simulink model "otonom_sim"  (R2021b)
settings: Solver=VariableStepAuto  StartTime=0.0  StopTime=50  RelTol=1e-3
libraries: sim3dautolib x2, slpidlib x1, robotmobilelib x1, simulink x1, sim3dlib x1
settings Model: Creator=Asus  LastModifiedBy=cx

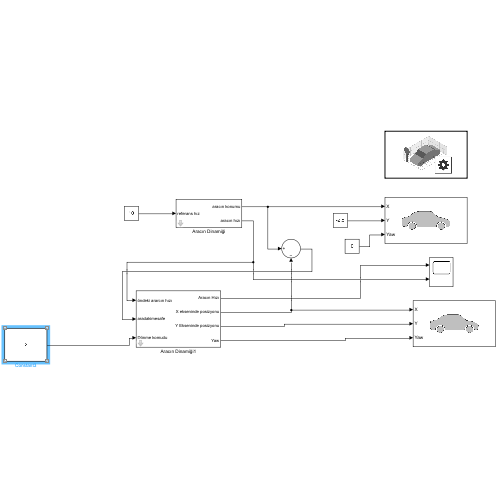
[thumbnail: Simulink's stored preview of the top-level diagram]
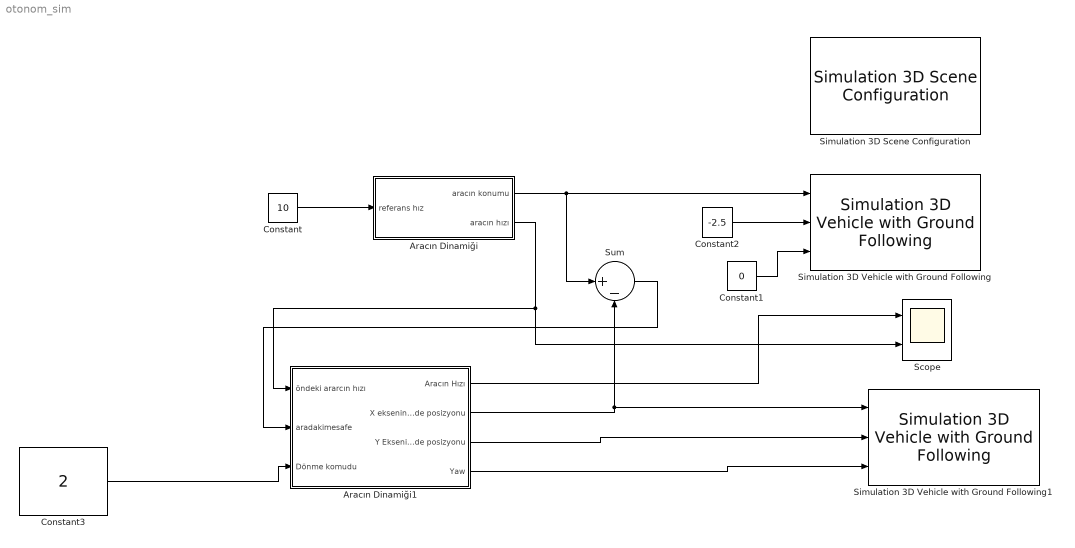
== system otonom_sim ==
  Aracın Dinamiği : Subsystem  mask{Konum=40, Hiz=20}
      mask prompts: Konum "Başlangıç Konumu"; Hiz "Başlangıç Hızı"
      mask TypeOptions Konum: başlangıç konumu/Value
      mask TypeOptions Hiz: başlangıç hızı/Value
  Aracın Dinamiği1 : Subsystem  mask{Konum=20, Hiz=40}
      mask prompts: Konum "Başlangıç Konumu"; Hiz "Başlangıç Hızı"
      mask TypeOptions Konum: başlangıç konumu/Value
      mask TypeOptions Hiz: başlangıç hızı/Value
  Constant : Constant  Value=10
  Constant1 : Constant  Value=0
  Constant2 : Constant  Value=-2.5
  Constant3 : Constant  Value=2
  Scope : Scope  NumInputPorts=2
  Simulation 3D Scene Configuration : sim3dlib/Simulation 3D Scene Configuration  Priority=0  ProjectFormat_internal=Default Scenes  ProjectFormat=Default Scenes  SceneDesc=Straight road  ProjectName=F:\MATLAB\R2021b\toolbox\shared\sim3d_projects\automotive_project\UE4\WindowsNoEditor\VehicleSimulation.exe  ScenePath=/Game/Maps/HwStrght  vehTagList={'Scene Origin';'SimulinkVehicle1';'SimulinkVehicle2'}  vehTag=SimulinkVehicle2  OpVisEn=off  Ts=0.1  EnableWindow=on  EnableWeather=off  SunAltitude=40.0  SunAzimuth=90  clouds=10  wind=1  fog=0  rain=0  sensorTag=MainCamera1  sensorId=1  sensorName=MainCamera1  mountLoc=Origin  offsetFlag=off  tmountOffset=[0, 0, 0]  rmountOffset=[0, 0, 0]  HorizontalResolution=1280  VerticalResolution=720  HorizontalFOV=60  mountPoint=[0 0 0]  mountOrientation=[0 0 0]  aMode=3  ID=1
      settings: SourceProductBaseCode=AE,DR,UV,VE
  Simulation 3D Vehicle with Ground Following : sim3dautolib/Simulation 3D Vehicle with Ground Following  Priority=-1  PassVehMesh=Muscle car  PassVehMesh_Internal=Muscle car  MeshPath=/MathWorksSimulation/Vehicles/Muscle/Meshes/SK_MuscleCar.SK_MuscleCar  TrackWidth=1.9  WheelBase=3  WheelRadius=0.35  VehColor=Blue  VehColor_Internal=Blue  InitialPos=[40, 0, 0]  InitialRot=[0, 0, 0]  ActorName=SimulinkVehicle1  SampleTime=0.1  ActorType=SimulinkVehicle  ID=1  aMode=3  ActorTag=SimulinkVehicle1  CoordinateScheme=ISO  VehLightsControl=off  HeadlightColor=[ 1, 1, 1 ]  HighBeamIntensity=100000  LowBeamIntensity=60000  HighBeamConeAngle=70  LowBeamConeAngle=70  LeftHeadlightOrientation=[ 0, 0 ]  RightHeadlightOrientation=[ 0, 0 ]  BrakelightIntensity=500  ReverselightIntensity=500  SignallightIntensity=500  SignallightPeriod=1  SignalPulseWidth=50  TransformOutportEnabled=off
      settings: SourceProductBaseCode=AE,DR,UV,VE
  Simulation 3D Vehicle with Ground Following1 : sim3dautolib/Simulation 3D Vehicle with Ground Following  Priority=-1  PassVehMesh=Muscle car  PassVehMesh_Internal=Muscle car  MeshPath=/MathWorksSimulation/Vehicles/Muscle/Meshes/SK_MuscleCar.SK_MuscleCar  TrackWidth=1.9  WheelBase=3  WheelRadius=0.35  VehColor=Red  VehColor_Internal=Red  InitialPos=[20, 0, 0]  InitialRot=[0, 0, 0]  ActorName=SimulinkVehicle2  SampleTime=0.1  ActorType=SimulinkVehicle  ID=2  aMode=3  ActorTag=SimulinkVehicle2  CoordinateScheme=ISO  VehLightsControl=off  HeadlightColor=[ 1, 1, 1 ]  HighBeamIntensity=100000  LowBeamIntensity=60000  HighBeamConeAngle=70  LowBeamConeAngle=70  LeftHeadlightOrientation=[ 0, 0 ]  RightHeadlightOrientation=[ 0, 0 ]  BrakelightIntensity=500  ReverselightIntensity=500  SignallightIntensity=500  SignallightPeriod=1  SignalPulseWidth=50  TransformOutportEnabled=off
      settings: SourceProductBaseCode=AE,DR,UV,VE
  Sum : Sum  Inputs=|+-
  wires:
  Constant/1 -> Aracın Dinamiği/1(referans hız)
  Aracın Dinamiği1/2(X ekseninde posizyonu) -> Sum/2, Simulation 3D Vehicle with Ground Following1/1
  Aracın Dinamiği1/3(Y Ekseninde posizyonu) -> Simulation 3D Vehicle with Ground Following1/2
  Aracın Dinamiği1/4(Yaw) -> Simulation 3D Vehicle with Ground Following1/3
  Constant1/1 -> Simulation 3D Vehicle with Ground Following/3
  Aracın Dinamiği/1(aracın konumu) -> Sum/1, Simulation 3D Vehicle with Ground Following/1
  Constant2/1 -> Simulation 3D Vehicle with Ground Following/2
  Aracın Dinamiği/2(aracın hızı) -> Scope/2, Aracın Dinamiği1/1(öndeki ararcın hızı)
  Sum/1 -> Aracın Dinamiği1/2(aradakimesafe)
  Aracın Dinamiği1/1(Aracın Hızı) -> Scope/1
  Constant3/1 -> Aracın Dinamiği1/3(Dönme komudu)

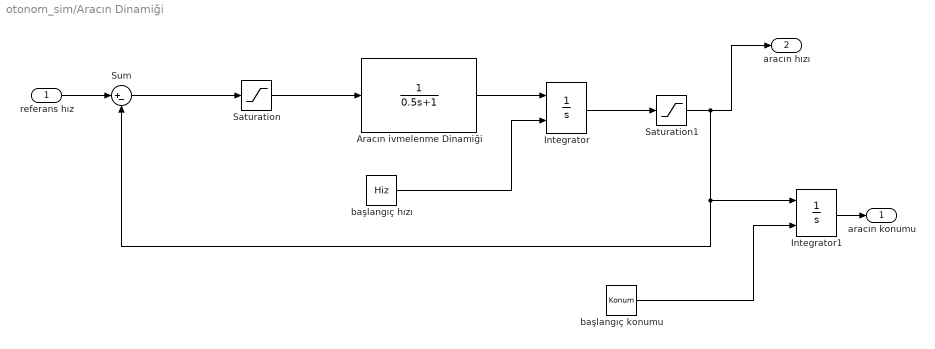
== system otonom_sim/Aracın Dinamiği ==
  referans hız : Inport
  Aracın ivmelenme Dinamiği : TransferFcn  Denominator=[0.5 1]
  Integrator : Integrator  InitialConditionSource=external
  Integrator1 : Integrator  InitialConditionSource=external
  Saturation : Saturate  UpperLimit=2  LowerLimit=-3
  Saturation1 : Saturate  UpperLimit=inf  LowerLimit=0
  Sum : Sum  Inputs=|+-
  başlangıç hızı : Constant  Value=Hiz
  başlangıç konumu : Constant  Value=Konum
  aracın konumu : Outport
  aracın hızı : Outport  Port=2
  wires:
  Sum/1 -> Saturation/1
  referans hız/1 -> Sum/1
  başlangıç konumu/1 -> Integrator1/2
  Saturation/1 -> Aracın ivmelenme Dinamiği/1
  Saturation1/1 -> aracın hızı/1, Integrator1/1, Sum/2
  başlangıç hızı/1 -> Integrator/2
  Integrator/1 -> Saturation1/1
  Aracın ivmelenme Dinamiği/1 -> Integrator/1
  Integrator1/1 -> aracın konumu/1

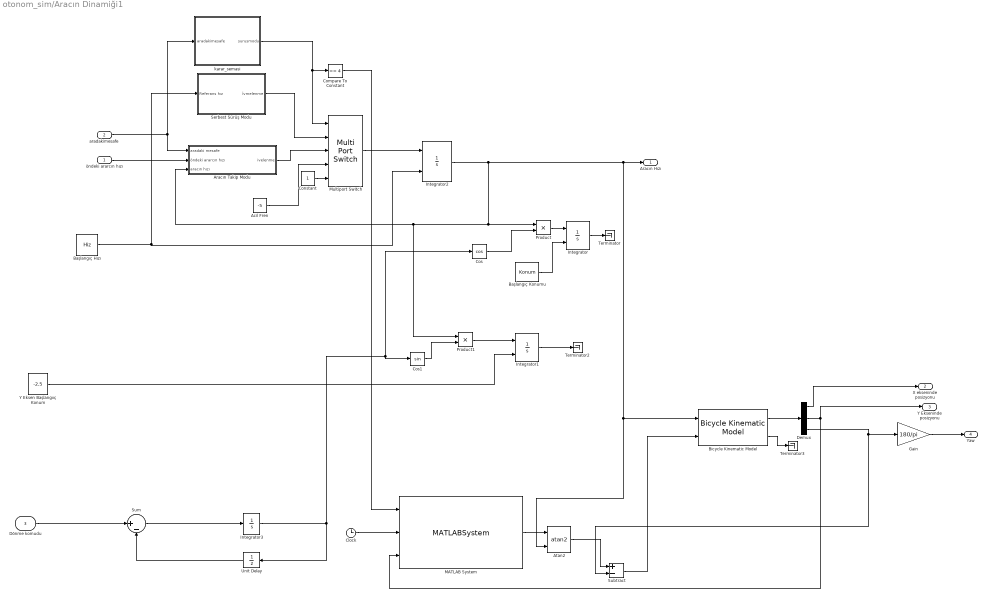
== system otonom_sim/Aracın Dinamiği1 ==
  öndeki ararcın hızı : Inport
  aradakimesafe : Inport  Port=2
  Dönme komudu : Inport  Port=3
  Acil Fren : Constant  Value=-5
  Aracın Takip Modu : Subsystem
  Atan2 : Trigonometry  Operator=atan2
  Başlangıç Hızı : Constant  Value=Hiz
  Başlangıç Konumu : Constant  Value=Konum
  Bicycle Kinematic Model : robotmobilelib/Bicycle Kinematic Model  VehicleInputs=Vehicle Speed & Steering Angle  WheelBase=3  VehicleSpeedRange=[0 12]  MaxSteeringAngle=pi/4  InitialState=[0; -3; 0]  SimulateUsing=Interpreted execution
      settings: SourceProductBaseCode=RO
  Clock : Clock
  Compare To Constant : simulink/Logic and Bit Operations/Compare To Constant  relop===  const=4  OutDataTypeStr=boolean
  Constant : Constant
  Cos : Trigonometry  Operator=cos
  Cos1 : Trigonometry
  Demux : Demux  Outputs=3
  Gain : Gain  Gain=180/pi
  Integrator : Integrator  InitialConditionSource=external
  Integrator1 : Integrator  InitialConditionSource=external
  Integrator2 : Integrator  InitialConditionSource=external  LimitOutput=on  UpperSaturationLimit=12  LowerSaturationLimit=0
  Integrator3 : Integrator
  MATLAB System : MATLABSystem  System=seritdegisimi  SimulateUsing=Interpreted execution
      mask Type: seritdegisimi
      mask Display:
      | disp('seritdegisimi');
      | port_label('input',1,'flag');
      | port_label('input',2,'clock');
      | port_label('input',3,'y');
      | port_label('output',1,'latSpeed');
  Multiport Switch : MultiPortSwitch  Inputs=4
  Product : Product
  Product1 : Product
  Serbest Sürüş Modu : Subsystem
  Subtract : Sum  Inputs=+-
  Sum : Sum  Inputs=|+-
  Terminator : Terminator
  Terminator2 : Terminator
  Terminator3 : Terminator
  Unit Delay : UnitDelay  SampleTime=-1  HasFrameUpgradeWarning=on
  Y Eksen Başlangııç Konum : Constant  Value=-2.5
  karar_semasi : Stateflow chart  TreatAsAtomicUnit=on
  Aracın Hızı : Outport
  X ekseninde posizyonu : Outport  Port=2
  Y Ekseninde posizyonu : Outport  Port=3
  Yaw : Outport  Port=4
  wires:
  öndeki ararcın hızı/1 -> Aracın Takip Modu/2(öndeki ararcın hızı)
  Integrator2/1 -> Product/1, Aracın Takip Modu/3(aracın hızı), Product1/1, Aracın Hızı/1, Atan2/2, Bicycle Kinematic Model/1
  aradakimesafe/1 -> karar_semasi/1(aradakimesafe), Aracın Takip Modu/1(aradaki mesafe)
  Aracın Takip Modu/1(ivelenme) -> Multiport Switch/3
  Serbest Sürüş Modu/1(İvmelenme) -> Multiport Switch/2
  karar_semasi/1(surusmodu) -> Compare To Constant/1, Multiport Switch/1
  Acil Fren/1 -> Multiport Switch/4
  Multiport Switch/1 -> Integrator2/1
  Başlangıç Hızı/1 -> Integrator2/2, Serbest Sürüş Modu/1(Referans hız)
  Cos/1 -> Product/2
  Product/1 -> Integrator/1
  Başlangıç Konumu/1 -> Integrator/2
  Integrator/1 -> Terminator/1
  Cos1/1 -> Product1/2
  Y Eksen Başlangııç Konum/1 -> Integrator1/2
  Integrator1/1 -> Terminator2/1
  Product1/1 -> Integrator1/1
  Dönme komudu/1 -> Sum/1
  Sum/1 -> Integrator3/1
  Unit Delay/1 -> Sum/2
  Integrator3/1 -> Unit Delay/1, Cos/1, Cos1/1
  Clock/1 -> MATLAB System/2
  Demux/1 -> X ekseninde posizyonu/1
  Gain/1 -> Yaw/1
  Demux/3 -> Subtract/2, Gain/1
  MATLAB System/1 -> Atan2/1
  Atan2/1 -> Subtract/1
  Subtract/1 -> Bicycle Kinematic Model/2
  Demux/2 -> Y Ekseninde posizyonu/1, MATLAB System/3
  Bicycle Kinematic Model/1 -> Demux/1
  Bicycle Kinematic Model/2 -> Terminator3/1
  Compare To Constant/1 -> MATLAB System/1
  Constant/1 -> Multiport Switch/5

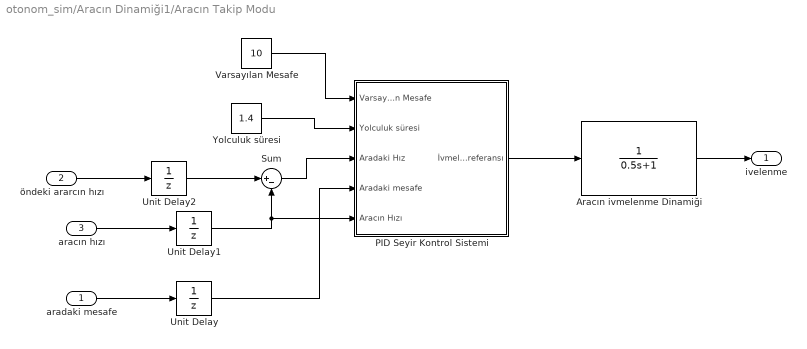
== system otonom_sim/Aracın Dinamiği1/Aracın Takip Modu ==
  aradaki mesafe : Inport
  öndeki ararcın hızı : Inport  Port=2
  aracın hızı : Inport  Port=3
  Aracın ivmelenme Dinamiği : TransferFcn  Denominator=[0.5 1]
  PID Seyir Kontrol Sistemi : Subsystem
  Sum : Sum  Inputs=|+-
  Unit Delay : UnitDelay  SampleTime=-1  HasFrameUpgradeWarning=on
  Unit Delay1 : UnitDelay  SampleTime=-1  HasFrameUpgradeWarning=on
  Unit Delay2 : UnitDelay  SampleTime=-1  HasFrameUpgradeWarning=on
  Varsayılan Mesafe : Constant  Value=10
  Yolculuk süresi : Constant  Value=1.4
  ivelenme : Outport
  wires:
  öndeki ararcın hızı/1 -> Unit Delay2/1
  Yolculuk süresi/1 -> PID Seyir Kontrol Sistemi/2(Yolculuk süresi)
  Aracın ivmelenme Dinamiği/1 -> ivelenme/1
  Unit Delay2/1 -> Sum/1
  PID Seyir Kontrol Sistemi/1(İvmelenme referansı) -> Aracın ivmelenme Dinamiği/1
  Varsayılan Mesafe/1 -> PID Seyir Kontrol Sistemi/1(Varsayılan Mesafe)
  Sum/1 -> PID Seyir Kontrol Sistemi/3(Aradaki Hız)
  aradaki mesafe/1 -> Unit Delay/1
  aracın hızı/1 -> Unit Delay1/1
  Unit Delay1/1 -> PID Seyir Kontrol Sistemi/5(Aracın Hızı), Sum/2
  Unit Delay/1 -> PID Seyir Kontrol Sistemi/4(Aradaki mesafe)

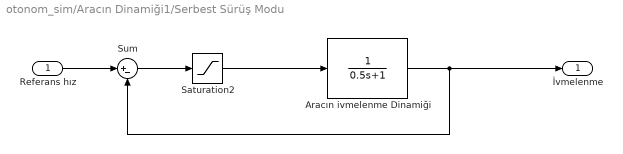
== system otonom_sim/Aracın Dinamiği1/Serbest Sürüş Modu ==
  Referans hız : Inport
  Aracın ivmelenme Dinamiği : TransferFcn  Denominator=[0.5 1]
  Saturation2 : Saturate  UpperLimit=2  LowerLimit=-3
  Sum : Sum  Inputs=|+-
  İvmelenme : Outport
  wires:
  Saturation2/1 -> Aracın ivmelenme Dinamiği/1
  Aracın ivmelenme Dinamiği/1 -> Sum/2, İvmelenme/1
  Referans hız/1 -> Sum/1
  Sum/1 -> Saturation2/1

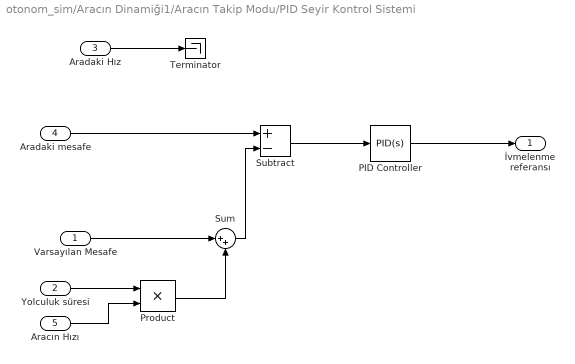
== system otonom_sim/Aracın Dinamiği1/Aracın Takip Modu/PID Seyir Kontrol Sistemi ==
  Varsayılan Mesafe : Inport
  Yolculuk süresi : Inport  Port=2
  Aradaki Hız : Inport  Port=3
  Aradaki mesafe : Inport  Port=4
  Aracın Hızı : Inport  Port=5
  PID Controller : slpidlib/PID Controller  Controller=PID  Form=Parallel  TimeDomain=Continuous-time  UseExternalTs=off  SampleTime=-1  IntegratorMethod=Forward Euler  FilterMethod=Forward Euler  ControllerParametersSource=internal  P=2  I=0.04  D=2.1  UseFilter=on  N=230  TunerSelectOption=Transfer Function Based (PID Tuner App)  InitialConditionSource=internal  InitialConditionForIntegrator=0  InitialConditionForFilter=0  DifferentiatorICPrevScaledInput=0  ExternalReset=none  TrackingMode=off  Kt=1  LimitOutput=on  SatLimitsSource=internal  UpperSaturationLimit=2  LowerSaturationLimit=-3  LinearizeAsGain=on  AntiWindupMode=clamping  Kb=1  POutMin=[]  POutMax=[]  IOutMin=[]  IOutMax=[]  DOutMin=[]  DOutMax=[]  NOutMin=[]  NOutMax=[]  SumOutMin=[]  SumOutMax=[]  SaturationOutMin=[]  SaturationOutMax=[]  PParamMin=[]  PParamMax=[]  IParamMin=[]  IParamMax=[]  DParamMin=[]  DParamMax=[]  NParamMin=[]  NParamMax=[]  KbParamMin=[]  KbParamMax=[]  KtParamMin=[]  KtParamMax=[]  KbOutMin=[]  KbOutMax=[]  KtOutMin=[]  KtOutMax=[]  IntegratorOutMin=[]  IntegratorOutMax=[]  FilterOutMin=[]  FilterOutMax=[]  SumI1OutMin=[]  SumI1OutMax=[]  SumI2OutMin=[]  SumI2OutMax=[]  SumI3OutMin=[]  SumI3OutMax=[]  SumI4OutMin=[]  SumI4OutMax=[]  SumDOutMin=[]  SumDOutMax=[]  DifferentiatorOutMin=[]  DifferentiatorOutMax=[]  FilterDiffOutCoefMin=[]  FilterDiffOutCoefMax=[]  ReciprocalOutMin=[]  ReciprocalOutMax=[]  SumDenOutMin=[]  SumDenOutMax=[]  SumNumOutMin=[]  SumNumOutMax=[]  DivideOutMin=[]  DivideOutMax=[]  UdiffTsProdOutMin=[]  UdiffTsProdOutMax=[]  NTsProdOutMin=[]  NTsProdOutMax=[]  UintegralTsProdOutMin=[]  UintegralTsProdOutMax=[]  UngainTsProdOutMin=[]  UngainTsProdOutMax=[]  IntegratorContinuousStateAttributes=''  IntegratorStateMustResolveToSignalObject=off  IntegratorRTWStateStorageClass=Auto  FilterContinuousStateAttributes=''  FilterStateMustResolveToSignalObject=off  FilterRTWStateStorageClass=Auto  ParallelPVariant=InternalParameters  IdealPVariant=Disabled  IVariant=InternalParameters  DVariant=InternalParameters  IntegratorVariant=Continuous  SatVariant=Enabled  AWVariant=ContClampingParallel  PCopyVariant=Disabled  TRVariant=Disabled  FdbkBlocksVariant=Forward  IdealPFdbkVariant=Disabled  SatFdbkVariant=Disabled  DerivativeFilterVariant=ContFilter  NVariant=InternalParameters  NCopyVariant=Disabled  FilterICVariant=InternalICsFilter  IntegratorICVariant=InternalICs  ExternalResetVariant=Disabled  TRSumVariant=Passthrough  SumFdbkVariant=Disabled  SumVariant=Sum_PID  TsampFilterVariant=InternalTs  TsampNgainVariant=Passthrough  TsampIntegralVariant=Passthrough  ExternalSaturationOutDataTypeStr=Inherit: Same as second input
  Product : Product
  Subtract : Sum  Inputs=+-
  Sum : Sum  Inputs=|++
  Terminator : Terminator
  İvmelenme referansı : Outport
  wires:
  Aracın Hızı/1 -> Product/2
  Yolculuk süresi/1 -> Product/1
  Varsayılan Mesafe/1 -> Sum/1
  Product/1 -> Sum/2
  Sum/1 -> Subtract/2
  Aradaki mesafe/1 -> Subtract/1
  Aradaki Hız/1 -> Terminator/1
  PID Controller/1 -> İvmelenme referansı/1
  Subtract/1 -> PID Controller/1

== stateflow chart otonom_sim/Aracın Dinamiği1/karar_semasi ==
  state SerbestSurusModu
    entry:
    surusmodu = 1;
  state AracTakipModu
    entry:
    surusmodu = 2;
  state donmemodu
    entry:
    surusmodu=4;
  state acilfren
    entry:
    surusmodu = 3;
  (default) -> SerbestSurusModu
  AracTakipModu -> SerbestSurusModu [order 1] : [aradakimesafe>50]
  SerbestSurusModu -> AracTakipModu [order 1] : [aradakimesafe>0 && aradakimesafe<=40]
  donmemodu -> SerbestSurusModu : [aradakimesafe < -30]
  SerbestSurusModu -> acilfren [order 2] : [aradakimesafe <= 10 && aradakimesafe > 0]
  AracTakipModu -> donmemodu [order 3] : [aradakimesafe<=30]
  acilfren -> AracTakipModu : [aradakimesafe>15]
  AracTakipModu -> acilfren [order 2] : [aradakimesafe<=10]
  data: surusmodu output; aradakimesafe input
